simulink model "PID_reduced"  (R2015b)
settings: Solver=VariableStepAuto  StartTime=0.0  StopTime=0.1  RelTol=1e-3
undefined symbols (not defined in the file): Jr, Kd_r, Ke, Ki_r, Kp_r, Kt, La, N, Ra, Tfv
settings Model: Creator=Erlingur  LastModifiedBy=Erlingur

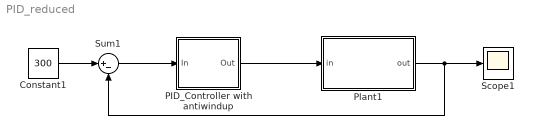
== system PID_reduced ==
  Constant1 : Constant  Value=300
  PID_Controller with antiwindup : Subsystem
  Plant1 : Subsystem
  Scope1 : Scope
  Sum1 : Sum  Inputs=|+-
  wires:
  PID_Controller with antiwindup/1(Out) -> Plant1/1(in)
  Plant1/1(out) -> Sum1/2, Scope1/1
  Constant1/1 -> Sum1/1
  Sum1/1 -> PID_Controller with antiwindup/1(In)

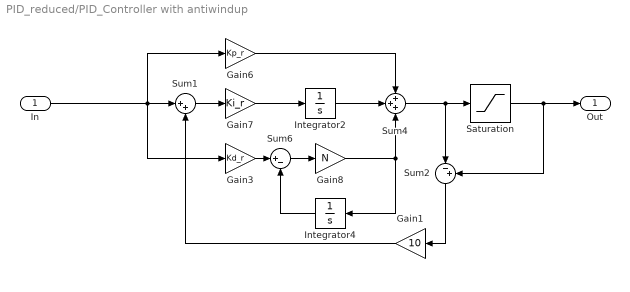
== system PID_reduced/PID_Controller with antiwindup ==
  In : Inport
  Gain1 : Gain  Gain=10
  Gain3 : Gain  Gain=Kd_r
  Gain6 : Gain  Gain=Kp_r
  Gain7 : Gain  Gain=Ki_r
  Gain8 : Gain  Gain=N
  Integrator2 : Integrator
  Integrator4 : Integrator
  Saturation : Saturate  UpperLimit=15  LowerLimit=-15
  Sum1 : Sum  Inputs=|++
  Sum2 : Sum  Inputs=|-+
  Sum4 : Sum  Inputs=+++
  Sum6 : Sum  Inputs=|+-
  Out : Outport
  wires:
  Gain7/1 -> Integrator2/1
  Integrator2/1 -> Sum4/2
  Gain6/1 -> Sum4/1
  In/1 -> Sum1/1, Gain3/1, Gain6/1
  Integrator4/1 -> Sum6/2
  Sum6/1 -> Gain8/1
  Gain8/1 -> Integrator4/1, Sum4/3
  Gain3/1 -> Sum6/1
  Sum4/1 -> Sum2/1, Saturation/1
  Saturation/1 -> Sum2/2, Out/1
  Sum1/1 -> Gain7/1
  Gain1/1 -> Sum1/2
  Sum2/1 -> Gain1/1

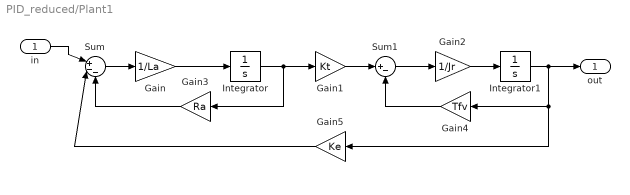
== system PID_reduced/Plant1 ==
  in : Inport
  Gain : Gain  Gain=1/La
  Gain1 : Gain  Gain=Kt
  Gain2 : Gain  Gain=1/Jr
  Gain3 : Gain  Gain=Ra
  Gain4 : Gain  Gain=Tfv
  Gain5 : Gain  Gain=Ke
  Integrator : Integrator
  Integrator1 : Integrator
  Sum : Sum  Inputs=|+--
  Sum1 : Sum  Inputs=|+-
  out : Outport
  wires:
  Sum1/1 -> Gain2/1
  Sum/1 -> Gain/1
  Integrator/1 -> Gain1/1, Gain3/1
  Gain/1 -> Integrator/1
  Gain2/1 -> Integrator1/1
  Gain3/1 -> Sum/3
  Integrator1/1 -> out/1, Gain5/1, Gain4/1
  Gain4/1 -> Sum1/2
  Gain1/1 -> Sum1/1
  in/1 -> Sum/1
  Gain5/1 -> Sum/2
